simulink model "test_RehaMove3_block__LowLevel1_simple"  (R2016b)
settings: Solver=FixedStepDiscrete  StartTime=0.0  StopTime=inf  FixedStep=0.05  RelTol=1e-3
libraries: LIB_RehaMove3 x1
settings Model: SimulationMode=external  ExtModeTrigDuration=10000  Creator=constantin  LastModifiedBy=valtin
settings DataIOCC: LimitDataPoints=on  SaveFormat=Array
settings OptimizationCC: ExpressionDepthLimit=2147483647  LifeSpan=1
settings DebuggingCC: UnderspecifiedInitializationDetection=Classic  MergeDetectMultiDrivingBlocksExec=none  SolverPrmCheckMsg=warning  StateNameClashWarn=warning  SFUnexpectedBacktrackingDiag=warning  SFNoUnconditionalDefaultTransitionDiag=warning  SFExecutionAtInitializationDiag=none
settings HardwareCC: ProdBitPerPointer=32  ProdBitPerSizeT=32  ProdBitPerPtrDiffT=32  ProdLargestAtomicFloat=None  ProdIntDivRoundTo=Undefined  ProdEndianess=Unspecified  ProdWordSize=32  ProdHWDeviceType=32-bit Generic
settings ModelReferenceCC: PropagateSignalLabelsOutOfModel=off
settings SFSimCC: SimParseCustomCode=off
settings RTWCC: SystemTargetFile=ert_linux.tlc  MakeCommand=make_rtw OPTS=-DWITH_HW OPTIMIZATION_FLAGS=-O3  TemplateMakefile=ert_linux.tmf  Description=Linux Embedded Coder  TargetLang=C++
settings CodeAppCC: IgnoreCustomStorageClasses=off  CustomSymbolStrType=$N$R$M  InternalIdentifier=Classic
settings STFCustomTargetCC: ModelReferenceCompliant=off  GeneratePreprocessorConditionals=Disable all  CombineOutputUpdateFcns=on  ERTCustomFileBanners=on  SupportComplex=off  RemoveResetFunc=on  SupportVariableSizeSignals=on  MATLABClassNameForMDSCustomization=Simulink.SoftwareTarget.ERTCustomization  GRTInterface=off  SystemTargetFile=ert_linux.tlc
settings ERTTargetCC: ModelReferenceCompliant=off  ParMdlRefBuildCompliant=off  CompOptLevelCompliant=off  ConcurrentExecutionCompliant=off  GeneratePreprocessorConditionals=Disable all  ERTFirstTimeCompliant=off  SupportComplex=off  SupportContinuousTime=on  SupportNonInlinedSFcns=on  SupportVariableSizeSignals=on  ModelStepFunctionPrototypeControlCompliant=off  CPPClassGenCompliant=off  UseToolchainInfoCompliant=off  ExtMode=on  MultiInstanceErrorCode=None  ERTCustomFileTemplate=ert_linux_file_process.tlc  ConvertIfToSwitch=off  SuppressUnreachableDefaultCases=off
settings ConfigComp: CovMetricSettings=dw  CovHtmlReporting=on  CovSaveCumulativeToWorkspaceVar=on  CovSaveSingleToWorkspaceVar=on  CovExternalEMLEnable=off  CovSFcnEnable=off
settings ConfigurationSet: Description=SimMechanics 2G

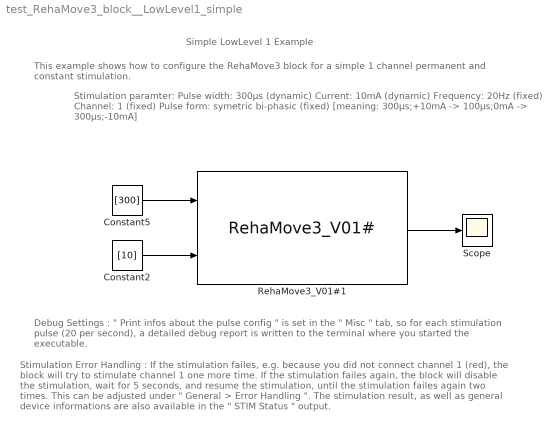
== system test_RehaMove3_block__LowLevel1_simple ==
  note: Stimulation Error Handling :
      | If the stimulation failes, e.g. because you did not connect channel 1 (red), the block will try to stimulate channel 1 one more time.
      | If the stimulation failes again, the block will disable the stimulation, wait for 5 seconds, and resume the stimulation,
      | until the stimulation failes again two times. This can be adjusted under " General > Error Handling ".
      | The stimulation result, as well as general device informations are also available in the " STIM Status " output.
  note: Debug Settings : " Print infos about the pulse config " is set in the " Misc " tab, so for each stimulation pulse (20 per second),
      | a detailed debug report is written to the terminal where you started the executable.
  note: Stimulation paramter:
      | Pulse width: 300µs (dynamic)
      | Current: 10mA (dynamic)
      | Frequency: 20Hz (fixed)
      | Channel: 1 (fixed)
      | Pulse form: symetric bi-phasic (fixed) [meaning: 300µs;+10mA -> 100µs;0mA -> 300µs;-10mA]
  note: This example shows how to configure the RehaMove3 block for a simple 1 channel permanent and constant stimulation.
  note: Simple LowLevel 1 Example
  Constant2 : Constant  Value=[10]  OutDataTypeStr=double  SampleTime=-1
  Constant5 : Constant  Value=[300]  OutDataTypeStr=double  SampleTime=-1
  RehaMove3_V01#1 : LIB_RehaMove3/RehaMove3_V01#  stimDevicePath=/dev/ttyUSB0  stimChannels=[ 1 ]  stimFrequency=20  stimRehaMoveProProtocol="Use the LowLevel protocol   -> Each stimulation pulse is send separatly."  stimMaxCurrent=90  stimMaxPulsWidth=500  stimBlockID=STIM1  stimTextSampleTime=0.05s (based on stimulation frequency)  SampleTime=0.05  stimThreadInit=on  stimThreadData=on  stimAbortError=2  stimTestAgain=5  llPulseShape=[0]  llNumberOfParts=1  llMaxStimVoltage=90V  llActivateDenervation=off  mlFStim=20  mlFStimDynamic=on  mlFKeepAlive=0.76923  mlUseSoftStart=on  mlUseRamps=off  mlRampsUpdates=3  mlRampsZeroUpdates=0  miscPrintBlockParam=off  miscPrintDeviceInfos=off  miscPrintSendInfos=off  miscPrintReceiveInfos=off  miscPrintInitInfos=off  miscPrintStimInfos=on  miscPrintRMPInitSettings=on  miscPrintCorrectionChargeWarnings=on  miscPrintSequenceErrors=on  miscPrintTimingErrors=on  miscUseColors=on  miscPrintStats=on  miscEnableAdvancedSettings=off  miscDisableVersionCheck=off
  Scope : Scope
  wires:
  RehaMove3_V01#1/1 -> Scope/1
  Constant5/1 -> RehaMove3_V01#1/1
  Constant2/1 -> RehaMove3_V01#1/2
